simulink model "jjk"  (Simulink 7.3)
settings: Solver=ode45  StartTime=0.0  StopTime=.9  RelTol=1e-3
libraries: powerlib_extras x2
settings Model: Creator=lap  LastModifiedBy=lap

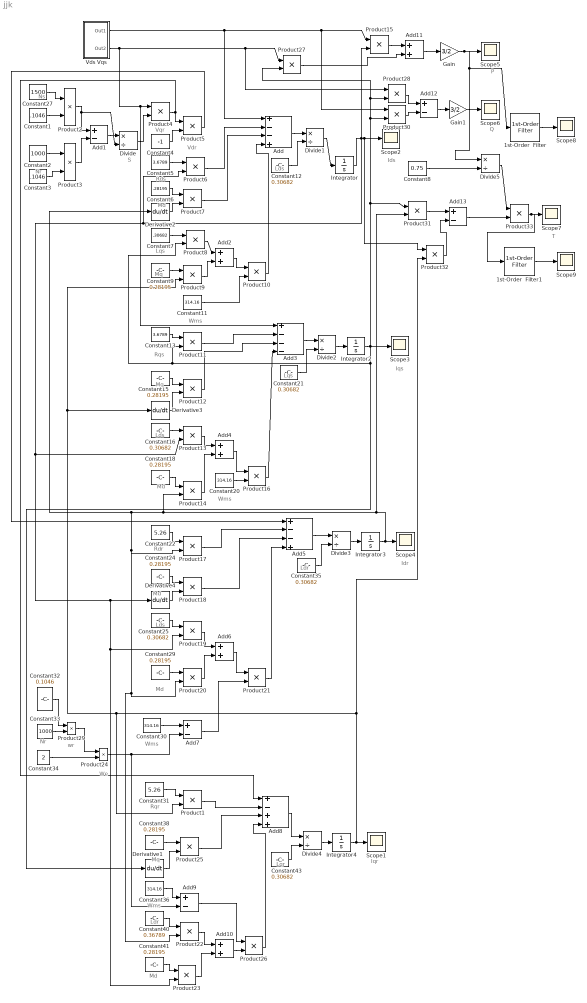
== system jjk ==
  note: Ns
  note: Nr
  note: S
  note: Vqr
  note: Vdr
  note: Rds
  note: Md
  note: Lqs
  note: Mq
  note: Wms
  note: Lds
  note: Ids
  note: Rqs
  note: Mq
  note: Lds
  note: Md
  note: Wms
  note: Lqs
  note: Iqs
  note: Rdr
  note: Md
  note: Lds
  note: Md
  note: Wms
  note: We
  note: wr
  note: Nr
  note: Ldr
  note: Idr
  note: Rqr
  note: Mq
  note: Wms
  note: Ldr
  note: Md
  note: Lqr
  note: Iqr
  note: P
  note: Q
  note: T
  1st-Order  Filter : powerlib_extras/Control  Blocks/1st-Order  Filter  DialogController=POWERSYS.PowerSysDialog  SystemSampleTime=-1  FilterType=Lowpass  Tc=12e-3  Initialize=off  Vac_Init=[0.8 -25 60]  Vdc_Init=-0.4  PlotResponse=off  param1=[1 500 1]
  1st-Order  Filter1 : powerlib_extras/Control  Blocks/1st-Order  Filter  DialogController=POWERSYS.PowerSysDialog  SystemSampleTime=-1  FilterType=Lowpass  Tc=12e-3  Initialize=off  Vac_Init=[0.8 -25 60]  Vdc_Init=-0.4  PlotResponse=off  param1=[1 500 1]
  Add : Sum  Inputs=+--+  OutDataType=fixdt(1, 16)  OutScaling=2^-10
  Add{1,7,9,12..13} (5 alike) : Sum  Inputs=+-  OutDataType=fixdt(1, 16)  OutScaling=2^-10
  Add{2,4,6,10..11} (5 alike) : Sum  OutDataType=fixdt(1, 16)  OutScaling=2^-10
  Add3 : Sum  Inputs=+---  OutDataType=fixdt(1, 16)  OutScaling=2^-10
  Add5 : Sum  Inputs=+--+  OutDataType=fixdt(1, 16)  OutScaling=2^-10
  Add8 : Sum  Inputs=+-++  OutDataType=fixdt(1, 16)  OutScaling=2^-10
  Constant1 : Constant  Value=.1046  OutDataType=fixdt(1, 16)  OutScaling=2^0
  Constant{11,20,30,36} (4 alike) : Constant  Value=314.16  OutDataType=fixdt(1, 16)  OutScaling=2^0
  Constant{12,16,21,25,35,43} (6 alike) : Constant  Value=0.30682  OutDataType=fixdt(1, 16)  OutScaling=2^0
  Constant13 : Constant  Value=3.6789  OutDataType=fixdt(1, 16)  OutScaling=2^0
  Constant{9,15,18,24,29,38,41} (7 alike) : Constant  Value=0.28195  OutDataType=fixdt(1, 16)  OutScaling=2^0
  Constant2 : Constant  Value=1000  OutDataType=fixdt(1, 16)  OutScaling=2^0
  Constant22 : Constant  Value=5.26  OutDataType=fixdt(1, 16)  OutScaling=2^0
  Constant27 : Constant  Value=1500  OutDataType=fixdt(1, 16)  OutScaling=2^0
  Constant3 : Constant  Value=.1046  OutDataType=fixdt(1, 16)  OutScaling=2^0
  Constant31 : Constant  Value=5.26  OutDataType=fixdt(1, 16)  OutScaling=2^0
  Constant32 : Constant  Value=0.1046  OutDataType=fixdt(1, 16)  OutScaling=2^0
  Constant33 : Constant  Value=1000  OutDataType=fixdt(1, 16)  OutScaling=2^0
  Constant34 : Constant  Value=2  OutDataType=fixdt(1, 16)  OutScaling=2^0
  Constant4 : Constant  Value=-1  OutDataType=fixdt(1, 16)  OutScaling=2^0
  Constant40 : Constant  Value=0.36789  OutDataType=fixdt(1, 16)  OutScaling=2^0
  Constant5 : Constant  Value=3.6789  OutDataType=fixdt(1, 16)  OutScaling=2^0
  Constant6 : Constant  Value=.28195  OutDataType=fixdt(1, 16)  OutScaling=2^0
  Constant7 : Constant  Value=.30682  OutDataType=fixdt(1, 16)  OutScaling=2^0
  Constant8 : Constant  Value=0.75  OutDataType=fixdt(1, 16)  OutScaling=2^0
  Derivative{1..4} (4 alike) : Derivative  LinearizePole=0.001
  Divide{,1..5} (6 alike) : Product  Inputs=*/  OutDataType=fixdt(1, 16)  OutScaling=2^-10
  Gain : Gain  Gain=3/2  ParameterDataType=fixdt(1, 16)  ParameterScaling=2^0  OutDataType=fixdt(1, 16)  OutScaling=2^0
  Gain1 : Gain  Gain=3/2  ParameterDataType=fixdt(1, 16)  ParameterScaling=2^0  OutDataType=fixdt(1, 16)  OutScaling=2^0
  Integrator : Integrator  LimitOutput=on
  Integrator2 : Integrator  LimitOutput=on  UpperSaturationLimit=20  LowerSaturationLimit=-20  ZeroCross=off
  Integrator3 : Integrator  LimitOutput=on  UpperSaturationLimit=20  LowerSaturationLimit=-20  ZeroCross=off
  Integrator4 : Integrator  LimitOutput=on  UpperSaturationLimit=20  LowerSaturationLimit=-20  ZeroCross=off
  Product{1..33} (33 alike) : Product  OutDataType=fixdt(1, 16)  OutScaling=2^0  RndMeth=Zero
  Scope{1..9} (9 alike) : Scope
      Scope1 settings: YMin=-20  YMax=20  SaveName=ScopeData4
      Scope2 settings: YMin=-20  YMax=20  SaveName=ScopeData5
      Scope3 settings: YMin=-20  YMax=20  SaveName=ScopeData6
      Scope4 settings: YMin=-20  YMax=20  SaveName=ScopeData7
      Scope5 settings: YMin=0  YMax=160  SaveName=ScopeData8
      Scope6 settings: YMin=-20  YMax=20  SaveName=ScopeData9
      Scope7 settings: YMin=-20  YMax=20  SaveName=ScopeData10
      Scope8 settings: YMin=0  YMax=160  SaveName=ScopeData11
      Scope9 settings: YMax=500  SaveName=ScopeData12
  Vds Vqs : Subsystem
  wires:
  Constant27/1 -> Product2/1
  Constant1/1 -> Product2/2
  Constant2/1 -> Product3/1
  Constant3/1 -> Product3/2
  Product2/1 -> Add1/1, Divide/2
  Product3/1 -> Add1/2
  Add1/1 -> Divide/1
  Vds Vqs/2(Out2) -> Product4/1, Add3/1, Product27/1, Product28/1
  Divide/1 -> Product4/2
  Product4/1 -> Product5/1, Add8/1
  Constant4/1 -> Product5/2
  Constant5/1 -> Product6/1
  Constant6/1 -> Product7/1
  Derivative2/1 -> Product7/2
  Constant7/1 -> Product8/1
  Product8/1 -> Add2/1
  Constant9/1 -> Product9/1
  Product9/1 -> Add2/2
  Add2/1 -> Product10/1
  Constant11/1 -> Product10/2
  Product6/1 -> Add/2
  Product7/1 -> Add/3
  Product10/1 -> Add/4
  Add/1 -> Divide1/1
  Constant12/1 -> Divide1/2
  Vds Vqs/1(Out1) -> Add/1, Product15/1, Product30/1
  Constant13/1 -> Product11/1
  Product11/1 -> Add3/2
  Constant15/1 -> Product12/1
  Derivative3/1 -> Product12/2
  Product12/1 -> Add3/3
  Constant16/1 -> Product13/1
  Product13/1 -> Add4/1
  Constant18/1 -> Product14/1
  Product14/1 -> Add4/2
  Add4/1 -> Product16/1
  Constant20/1 -> Product16/2
  Product16/1 -> Add3/4
  Add3/1 -> Divide2/1
  Constant21/1 -> Divide2/2
  Divide2/1 -> Integrator2/1
  Integrator2/1 -> Scope3/1, Derivative1/1, Product11/2, Product8/2, Product27/2, Product28/2, Product30/2, Product31/1
  Product5/1 -> Add5/1
  Constant22/1 -> Product17/1
  Product17/1 -> Add5/2
  Constant24/1 -> Product18/1
  Derivative4/1 -> Product18/2
  Constant25/1 -> Product19/1
  Product19/1 -> Add6/1
  Constant29/1 -> Product20/1
  Product20/1 -> Add6/2
  Constant34/1 -> Product24/2
  Constant32/1 -> Product29/1
  Product29/1 -> Product24/1
  Constant33/1 -> Product29/2
  Product24/1 -> Add7/2, Add9/2
  Constant30/1 -> Add7/1
  Add6/1 -> Product21/1
  Add7/1 -> Product21/2
  Product18/1 -> Add5/3
  Product21/1 -> Add5/4
  Add5/1 -> Divide3/1
  Constant35/1 -> Divide3/2
  Divide3/1 -> Integrator3/1
  Integrator3/1 -> Scope4/1, Product14/2, Product17/2, Product20/2, Product22/2, Derivative2/1, Product31/2
  Constant31/1 -> Product1/1
  Product1/1 -> Add8/2
  Constant38/1 -> Product25/1
  Derivative1/1 -> Product25/2
  Constant36/1 -> Add9/1
  Constant40/1 -> Product22/1
  Constant41/1 -> Product23/1
  Product22/1 -> Add10/1
  Product23/1 -> Add10/2
  Add9/1 -> Product26/1
  Add10/1 -> Product26/2
  Divide4/1 -> Integrator4/1
  Integrator4/1 -> Scope1/1, Product1/2, Product9/2, Derivative3/1, Product32/2
  Product25/1 -> Add8/3
  Product26/1 -> Add8/4
  Add8/1 -> Divide4/1
  Constant43/1 -> Divide4/2
  Product15/1 -> Add11/1
  Product27/1 -> Add11/2
  Add11/1 -> Gain/1
  Gain/1 -> Scope5/1, Divide5/1, 1st-Order  Filter/1
  Product28/1 -> Add12/1
  Product30/1 -> Add12/2
  Add12/1 -> Gain1/1
  Gain1/1 -> Scope6/1
  Constant8/1 -> Divide5/2
  Product31/1 -> Add13/1
  Product32/1 -> Add13/2
  Divide5/1 -> Product33/1
  Add13/1 -> Product33/2
  Product33/1 -> Scope7/1, 1st-Order  Filter1/1
  1st-Order  Filter1/1 -> Scope9/1
  Divide1/1 -> Integrator/1
  Integrator/1 -> Product6/2, Product13/2, Derivative4/1, Product19/2, Product23/2, Product15/2, Scope2/1, Product32/1
  1st-Order  Filter/1 -> Scope8/1

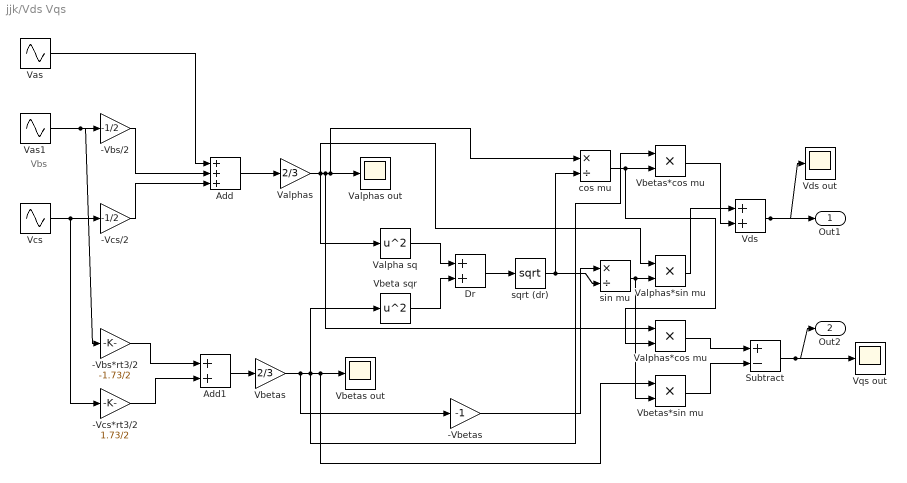
== system jjk/Vds Vqs ==
  note: Vbs
  "-Vbetas " : Gain  Gain=-1  ParameterDataType=fixdt(1, 16)  ParameterScaling=2^0  OutDataType=fixdt(1, 16)  OutScaling=2^0
  -Vbs*rt3/2 : Gain  Gain=-1.73/2  ParameterDataType=fixdt(1, 16)  ParameterScaling=2^0  OutDataType=fixdt(1, 16)  OutScaling=2^0
  -Vbs/2 : Gain  Gain=-1/2  ParameterDataType=fixdt(1, 16)  ParameterScaling=2^0  OutDataType=fixdt(1, 16)  OutScaling=2^0
  -Vcs*rt3/2 : Gain  Gain=1.73/2  ParameterDataType=fixdt(1, 16)  ParameterScaling=2^0  OutDataType=fixdt(1, 16)  OutScaling=2^0
  -Vcs/2 : Gain  Gain=-1/2  ParameterDataType=fixdt(1, 16)  ParameterScaling=2^0  OutDataType=fixdt(1, 16)  OutScaling=2^0
  Add : Sum  Inputs=+++  OutDataType=fixdt(1, 16)  OutScaling=2^-10
  Add1 : Sum  OutDataType=fixdt(1, 16)  OutScaling=2^-10
  Dr : Sum  OutDataType=fixdt(1, 16)  OutScaling=2^-10
  Subtract : Sum  Inputs=+-  OutDataType=fixdt(1, 16)  OutScaling=2^-10
  Valpha sq : Math  Operator=square  OutDataType=fixdt(1, 16)  OutScaling=2^0  SaturateOnIntegerOverflow=on
  Valphas : Gain  Gain=2/3  ParameterDataType=fixdt(1, 16)  ParameterScaling=2^0  OutDataType=fixdt(1, 16)  OutScaling=2^0
  Valphas out : Scope
  Valphas*cos mu : Product  OutDataType=fixdt(1, 16)  OutScaling=2^0  RndMeth=Zero
  Valphas*sin mu : Product  OutDataType=fixdt(1, 16)  OutScaling=2^0  RndMeth=Zero
  Vas : Sin  Amplitude=230  Bias=0  Frequency=314  Phase=0  Samples=10  SampleTime=0  Offset=0
  Vas1 : Sin  Amplitude=230  Bias=0  Frequency=314  Phase=-2.09  Samples=10  SampleTime=0  Offset=0
  Vbeta sqr : Math  Operator=square  OutDataType=fixdt(1, 16)  OutScaling=2^0  SaturateOnIntegerOverflow=on
  Vbetas : Gain  Gain=2/3  ParameterDataType=fixdt(1, 16)  ParameterScaling=2^0  OutDataType=fixdt(1, 16)  OutScaling=2^0
  Vbetas out : Scope
      settings: YMin=-300  YMax=300
  Vbetas*cos mu : Product  OutDataType=fixdt(1, 16)  OutScaling=2^0  RndMeth=Zero
  Vbetas*sin mu : Product  OutDataType=fixdt(1, 16)  OutScaling=2^0  RndMeth=Zero
  Vcs : Sin  Amplitude=230  Bias=0  Frequency=314  Phase=-4.18  Samples=10  SampleTime=0  Offset=0
  Vds : Sum  OutDataType=fixdt(1, 16)  OutScaling=2^-10
  Vds out : Scope
      settings: YMin=-300  YMax=300  SaveName=ScopeData2
  Vqs out : Scope
      settings: YMin=220  YMax=229  SaveName=ScopeData3
  cos mu : Product  Inputs=*/  OutDataType=fixdt(1, 16)  OutScaling=2^-10
  sin mu : Product  Inputs=*/  OutDataType=fixdt(1, 16)  OutScaling=2^-10
  sqrt (dr) : Math  Operator=sqrt  OutDataType=fixdt(1, 16)  OutScaling=2^0  SaturateOnIntegerOverflow=on
  Out1 : Outport
  Out2 : Outport  Port=2
  wires:
  Vas1/1 -> -Vbs/2/1, -Vbs*rt3/2/1
  Vcs/1 -> -Vcs/2/1, -Vcs*rt3/2/1
  Vas/1 -> Add/1
  -Vbs/2/1 -> Add/2
  -Vcs/2/1 -> Add/3
  Add/1 -> Valphas/1
  -Vbs*rt3/2/1 -> Add1/1
  -Vcs*rt3/2/1 -> Add1/2
  Add1/1 -> Vbetas/1
  Valphas/1 -> Valpha sq/1, Valphas*sin mu/1, Valphas out/1, cos mu/1, Valphas*cos mu/1
  Vbetas/1 -> Vbeta sqr/1, Vbetas*cos mu/1, Vbetas*sin mu/1, Vbetas out/1, "-Vbetas "/1
  Valpha sq/1 -> Dr/1
  Vbeta sqr/1 -> Dr/2
  Dr/1 -> sqrt (dr)/1
  "-Vbetas "/1 -> sin mu/1
  sqrt (dr)/1 -> sin mu/2, cos mu/2
  sin mu/1 -> Valphas*sin mu/2, Vbetas*sin mu/2
  cos mu/1 -> Vbetas*cos mu/2, Valphas*cos mu/2
  Valphas*sin mu/1 -> Vds/1
  Vbetas*cos mu/1 -> Vds/2
  Vds/1 -> Vds out/1, Out1/1
  Valphas*cos mu/1 -> Subtract/1
  Subtract/1 -> Vqs out/1, Out2/1
  Vbetas*sin mu/1 -> Subtract/2
